simulink model "Transformation_V11"  (R2018a)
settings: Solver=FixedStepDiscrete  StartTime=0.0  StopTime=10.0  RelTol=1e-3
InitFcn:
  | Ts_xadc = 0.1;
values from neighbouring files (symbols this model uses):
  T_mech = 2e-08    [TransformationSkript.m]
libraries: hdlsllib x14, simulink x8, simulink_need_slupdate x1
(part 1 of 4)
settings Model: DataTypeOverride=Off  Creator=trichte  LastModifiedBy=Wendel
settings DataIOCC: LimitDataPoints=on  SaveFormat=Array  SaveOutput=off  SaveTime=off
settings OptimizationCC: BlockReduction=off  ConditionallyExecuteInputs=off  DefaultParameterBehavior=Inlined  LifeSpan=inf
settings DebuggingCC: AlgebraicLoopMsg=error  SolverPrmCheckMsg=warning  SingleTaskRateTransMsg=error  AllowSymbolicDim=off  StrictBusMsg=ErrorOnBusTreatedAsVector  SFUnexpectedBacktrackingDiag=warning  SFNoUnconditionalDefaultTransitionDiag=warning  SFExecutionAtInitializationDiag=none
settings HardwareCC: ProdBitPerPointer=32  ProdBitPerSizeT=32  ProdBitPerPtrDiffT=32  ProdLargestAtomicFloat=None  ProdIntDivRoundTo=Undefined  ProdEndianess=Unspecified  ProdWordSize=32  ProdHWDeviceType=ASIC/FPGA->ASIC/FPGA  ProdEqTarget=off
settings ModelReferenceCC: PropagateSignalLabelsOutOfModel=off
settings CodeAppCC: StateflowObjectComments=on
settings GRTTargetCC: TargetLangStandard=C89/C90 (ANSI)  GeneratePreprocessorConditionals=Disable all
settings ConfigComp: CovMetricSettings=dw  CovHtmlReporting=on  CovSaveCumulativeToWorkspaceVar=on  CovSaveSingleToWorkspaceVar=on  CovExternalEMLEnable=off  CovSFcnEnable=off

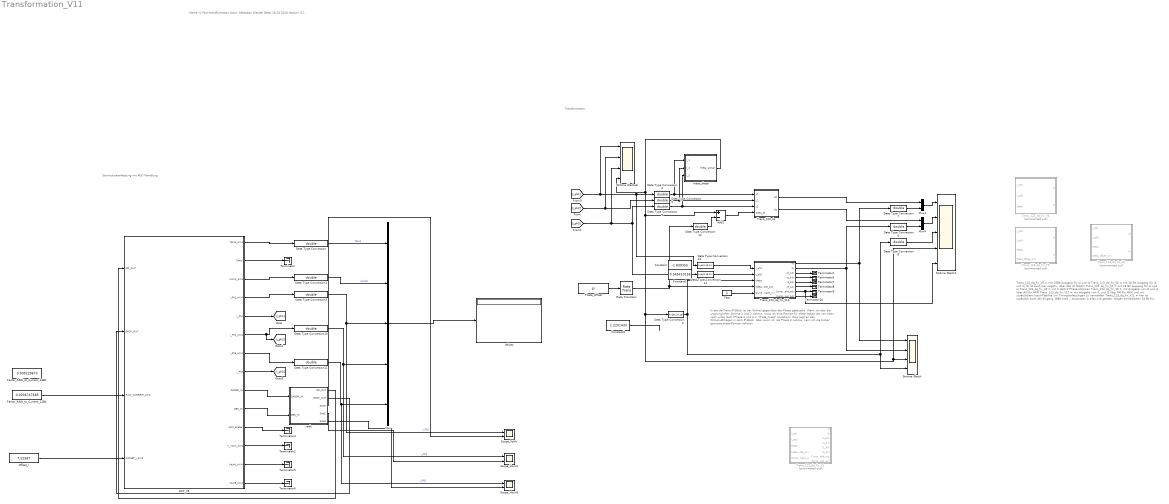
== system Transformation_V11 ==
  note: Trans_123_dq_fix_V5 = mit 16Bit Ausgang für id und iq
      | Trans_123_dq_fix_V6 = mit 18 Bit Ausgang für id und iq (iq ist auch hier negativ, aber das ist falsch)
      | Trans_123_dq_fix_V7 = mit 18 Bit Ausgang für id und iq
      | Trans_123_dq_fix_V8 = mit 3 statt 2 Phasenströmen
      | Trans_123_dq_fix_V9 = mit Ausgabe von id und iq über AXI für ARM
      | Trans_123_dq_fix_V10 = mit Ausgabe von i1 und i3 über AXI für ARM und mit zusätzlichem Input-Pipeline um Timingverletzungen zu vermeiden
      | Trans_123_dq_fix_V11 = hier ist zusätzlich auch der Eingang 18Bit breit
      |
      | ...ansonsten is alles wie gehabt. Wegen einheitlichen 18 Bit für alle Größem wird jedoch 18 Bit genutzt!
  note: Stromistwererfassung mit ADC-Wandlung
  note: Transformation
  note: In der dq-Trans-IP-Block ist der Winkel gegenüber der Phase getauscht.
      | Wenn ich also die ursprünglichen Ströme 1 und 2 nehme,
      |  muss ich eine Rampe für theta haben die von oben nach unten läuft
      | (Phase 2 und 3 in "theta_meas" tauschen).
      | Dies liegt an den Winkel-Abfragen in dem IP-Block.
      | Aber wenn ich die Phase 3 nehme, kann ich die bisher genutzte theta-Rampe nehmen.
  note: Clarke- & Park-transformation
      |
      | Autor: Sebastian Wendel
      | Date: 26.03.2018
      | Version: 0.1
  Add1 : Sum  Inputs=+-  OutDataTypeStr=Inherit: Same as accumulator
  Constant : Constant  Value=-1.839355
  Constant1 : Constant  Value=0.545410156
  Constant2 : Constant  Value=1.2201433
  DUT_V5 : Subsystem  TreatAsAtomicUnit=on
  Data Type Conversion{,1,3..12} (12 alike) : DataTypeConversion  OutDataTypeStr=double
  Data Type Conversion13 : DataTypeConversion  OutDataTypeStr=fixdt(1,18,11)
  Data Type Conversion14 : DataTypeConversion  OutDataTypeStr=fixdt(1,18,11)
  Data Type Conversion2 : DataTypeConversion  OutDataTypeStr=fixdt(1,24,20)
  Factor_RAW_to_Current_12Bit : Constant  Value=0.0036747685  OutDataTypeStr=fixdt(0,24,24)
  Factor_RAW_to_Current_16Bit : Constant  Value=0.000229673  OutDataTypeStr=fixdt(0,24,24)
  Mux : Mux  Inputs=5
  Mux3 : Mux  Inputs=2
  Mux4 : Mux  Inputs=2
  Offset_i : Constant  Value=7.52587  OutDataTypeStr=fixdt(0,16,11)
  Rate Transition : RateTransition  OutPortSampleTime=T_mech
  Scope_Vaux0 : Scope  NumInputPorts=2
  Scope_Vaux8 : Scope  NumInputPorts=2
  Scope_VpVn : Scope  NumInputPorts=2
  Ströme Gleich : Scope  NumInputPorts=4
  Ströme Gleich1 : Scope  NumInputPorts=5
  Ströme Wechsel : Scope  NumInputPorts=4
  Terminator{,1..10} (11 alike) : Terminator
  Test : Constant  OutDataTypeStr=boolean  SampleTime=T_mech
  Theta_Offset : Constant  Value=pi  OutDataTypeStr=fixdt(1,24,20)
  Trans_123_dq : Subsystem
  Trans_123_dq_fix_V1 : Subsystem  Commented=on  TreatAsAtomicUnit=on
  Trans_123_dq_fix_V11 : Subsystem  TreatAsAtomicUnit=on
  Trans_123_dq_fix_V3 : Subsystem  Commented=on  TreatAsAtomicUnit=on
  Trans_123_dq_fix_V5 : Subsystem  Commented=on  TreatAsAtomicUnit=on
  Trans_123_dq_fix_V6 : Subsystem  Commented=on  TreatAsAtomicUnit=on
  Values : Display
      settings: Format=hex (Stored Integer)
  meas_theta : Subsystem
  xadc : Subsystem
  wires:
  DUT_V5/1(Temp_AXI4) -> Data Type Conversion/1
  DUT_V5/3(VccInt_AXI4) -> Data Type Conversion1/1
  DUT_V5/4(i_Ph1_AXI4) -> Data Type Conversion3/1
  DUT_V5/7(i_Ph3_AXI4) -> Data Type Conversion11/1
  DUT_V5/6(i_Ph2_AXI4) -> [i_ph2], Data Type Conversion10/1
  Mux/1 -> Values/1
  Data Type Conversion/1 -> Mux/1  "Temp"
  Data Type Conversion3/1 -> Scope_VpVn/1, Mux/3  "i_Ph1"
  Data Type Conversion10/1 -> Scope_Vaux0/1, Mux/4  "i_Ph2"
  Data Type Conversion11/1 -> Scope_Vaux8/1, Mux/5  "i_Ph3"
  Data Type Conversion1/1 -> Mux/2  "VccInt"
  DUT_V5/9(DADDR_IN) -> xadc/1(DADDR_IN)
  DUT_V5/10(DEN_IN) -> xadc/2(DEN_IN)
  xadc/2(DRDY_OUT) -> DUT_V5/2(DRDY_OUT)
  xadc/1(DO_OUT) -> DUT_V5/1(DO_OUT)
  DUT_V5/2(Temp) -> Terminator/1
  DUT_V5/11(ADC_enable) -> Terminator4/1
  Factor_RAW_to_Current_12Bit/1 -> DUT_V5/3(RAW_CURRENT_AXI4)
  Offset_i/1 -> DUT_V5/4(OFFSET_I_AXI4)
  DUT_V5/12(V_VpVn_AXI4) -> Terminator2/1
  DUT_V5/13(Vaux0_AXI4) -> Terminator5/1
  DUT_V5/14(Vaux8_AXI4) -> Terminator6/1
  xadc/3(Sine1) -> Scope_VpVn/2
  xadc/4(Sine2) -> Scope_Vaux0/2
  xadc/5(Sine3) -> Scope_Vaux8/2
  Data Type Conversion2/1 -> Trans_123_dq_fix_V11/3(theta), Ströme Gleich/4, Data Type Conversion8/1
  Trans_123_dq/1(Ud) -> Mux3/1
  Trans_123_dq/2(Uq) -> Mux4/1
  Mux3/1 -> Ströme Gleich1/1
  Data Type Conversion7/1 -> Mux3/2
  Data Type Conversion6/1 -> Mux4/2
  Mux4/1 -> Ströme Gleich1/2
  Data Type Conversion8/1 -> Ströme Gleich1/3
  meas_theta/1(theta_arctan) -> Ströme Wechsel/4, Data Type Conversion2/1, Ströme Gleich/3, Ströme Gleich1/4, Add1/1
  Data Type Conversion4/1 -> meas_theta/1(I_1), Trans_123_dq/1(L1)
  Data Type Conversion9/1 -> meas_theta/3(I_3), Trans_123_dq/3(L3)
  Data Type Conversion5/1 -> meas_theta/2(I_2), Trans_123_dq/2(L2)
  DUT_V5/5(i_Ph1) -> [i_ph1]
  DUT_V5/8(i_Ph3) -> [i_ph3]
  [i_ph2] -> Ströme Wechsel/2, Data Type Conversion5/1
  Trans_123_dq_fix_V11/1(id) -> Ströme Gleich/1, Data Type Conversion7/1
  Trans_123_dq_fix_V11/2(iq) -> Ströme Gleich/2, Data Type Conversion6/1
  Theta_Offset/1 -> Rate Transition/1
  Data Type Conversion12/1 -> Add1/2
  Add1/1 -> Trans_123_dq/4(theta_el)
  Trans_123_dq_fix_V11/4(iq_AXI) -> Terminator3/1
  Trans_123_dq_fix_V11/3(id_AXI) -> Terminator1/1
  Rate Transition/1 -> Data Type Conversion12/1, Trans_123_dq_fix_V11/4(theta_offset_AXI)
  Trans_123_dq_fix_V11/5(i1_AXI) -> Terminator7/1
  Trans_123_dq_fix_V11/6(i3_AXI) -> Terminator8/1
  Data Type Conversion13/1 -> Trans_123_dq_fix_V11/1(i_ph1)
  Data Type Conversion14/1 -> Trans_123_dq_fix_V11/2(i_ph3)
  Trans_123_dq_fix_V11/7(CurrentValid_out) -> Ströme Gleich1/5, Terminator9/1
  Test/1 -> Trans_123_dq_fix_V11/5(CurrentValid_in)
  Trans_123_dq_fix_V11/8(CurrentValid_out_AXI) -> Terminator10/1
  [i_ph1] -> Ströme Wechsel/1, Data Type Conversion13/1, Data Type Conversion4/1
  [i_ph3] -> Ströme Wechsel/3, Data Type Conversion14/1, Data Type Conversion9/1
  Constant2/1 -> ?

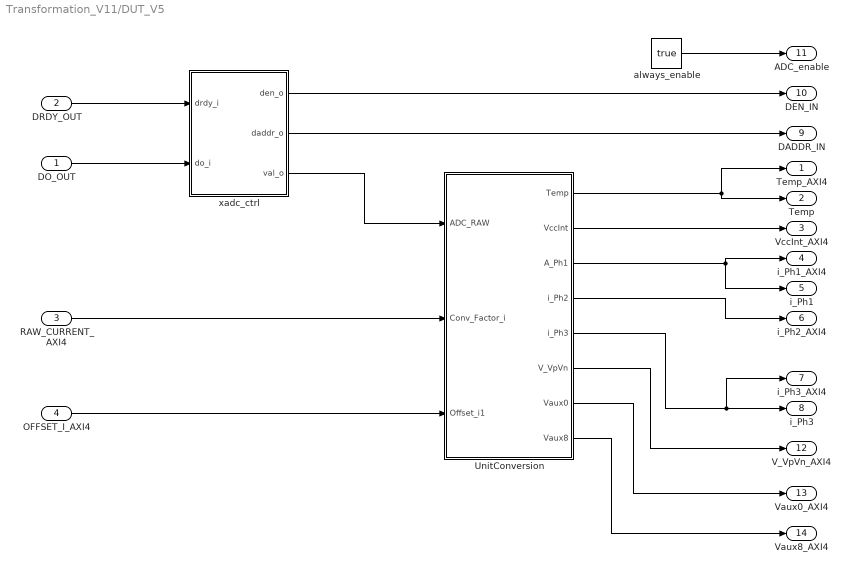
== system Transformation_V11/DUT_V5 ==
  DO_OUT : Inport
  DRDY_OUT : Inport  Port=2
  RAW_CURRENT_AXI4 : Inport  Port=3
  OFFSET_I_AXI4 : Inport  Port=4
  UnitConversion : Subsystem
  always_enable : Constant  Value=true  OutDataTypeStr=boolean
  xadc_ctrl : MATLAB Function  TreatAsAtomicUnit=on
  Temp_AXI4 : Outport
  Temp : Outport  Port=2
  VccInt_AXI4 : Outport  Port=3
  i_Ph1_AXI4 : Outport  Port=4
  i_Ph1 : Outport  Port=5
  i_Ph2_AXI4 : Outport  Port=6
  i_Ph3_AXI4 : Outport  Port=7
  i_Ph3 : Outport  Port=8
  DADDR_IN : Outport  Port=9
  DEN_IN : Outport  Port=10
  ADC_enable : Outport  Port=11
  V_VpVn_AXI4 : Outport  Port=12
  Vaux0_AXI4 : Outport  Port=13
  Vaux8_AXI4 : Outport  Port=14
  wires:
  xadc_ctrl/3(val_o) -> UnitConversion/1(ADC_RAW)
  UnitConversion/5(i_Ph3) -> i_Ph3/1, i_Ph3_AXI4/1
  UnitConversion/3(A_Ph1) -> i_Ph1/1, i_Ph1_AXI4/1
  UnitConversion/4(i_Ph2) -> i_Ph2_AXI4/1
  UnitConversion/2(VccInt) -> VccInt_AXI4/1
  UnitConversion/1(Temp) -> Temp/1, Temp_AXI4/1
  DRDY_OUT/1 -> xadc_ctrl/1(drdy_i)
  DO_OUT/1 -> xadc_ctrl/2(do_i)
  xadc_ctrl/1(den_o) -> DEN_IN/1
  xadc_ctrl/2(daddr_o) -> DADDR_IN/1
  always_enable/1 -> ADC_enable/1
  RAW_CURRENT_AXI4/1 -> UnitConversion/2(Conv_Factor_i)
  UnitConversion/6(V_VpVn) -> V_VpVn_AXI4/1
  OFFSET_I_AXI4/1 -> UnitConversion/3(Offset_i1)
  UnitConversion/7(Vaux0) -> Vaux0_AXI4/1
  UnitConversion/8(Vaux8) -> Vaux8_AXI4/1

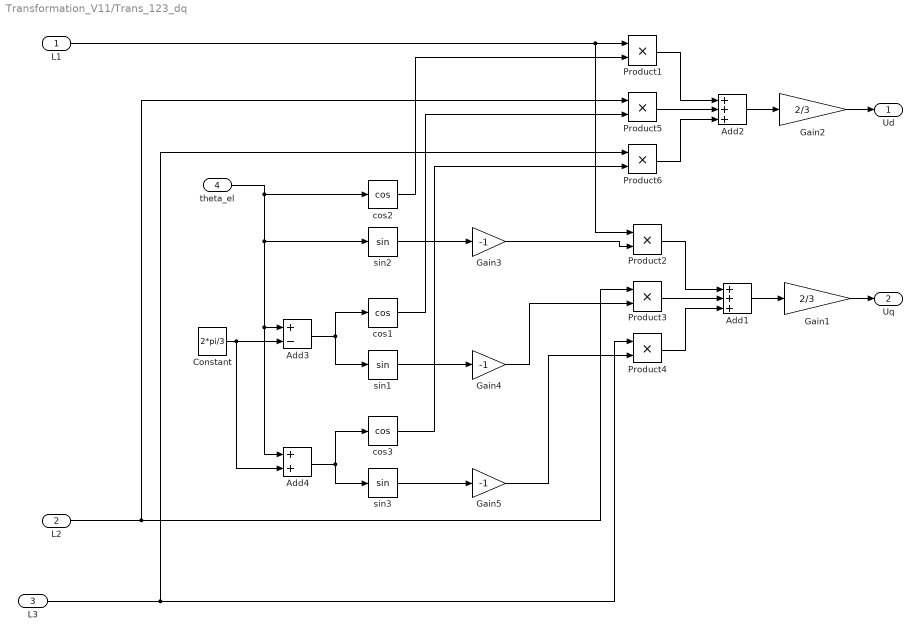
== system Transformation_V11/Trans_123_dq ==
  L1 : Inport
  L2 : Inport  Port=2
  L3 : Inport  Port=3
  theta_el : Inport  Port=4
  Add1 : Sum  Inputs=+++
  Add2 : Sum  Inputs=+++
  Add3 : Sum  Inputs=+-
  Add4 : Sum
  Constant : Constant  Value=2*pi/3  SampleTime=T_mech
  Gain1 : Gain  Gain=2/3
  Gain2 : Gain  Gain=2/3
  Gain3 : Gain  Gain=-1
  Gain4 : Gain  Gain=-1
  Gain5 : Gain  Gain=-1
  Product{1..6} (6 alike) : Product  RndMeth=Zero
  cos1 : Trigonometry  Operator=cos
  cos2 : Trigonometry  Operator=cos
  cos3 : Trigonometry  Operator=cos
  sin1 : Trigonometry
  sin2 : Trigonometry
  sin3 : Trigonometry
  Ud : Outport
  Uq : Outport  Port=2
  wires:
  Gain5/1 -> Product4/2
  Gain4/1 -> Product3/2
  Gain3/1 -> Product2/2
  sin3/1 -> Gain5/1
  sin1/1 -> Gain4/1
  sin2/1 -> Gain3/1
  L3/1 -> Product4/1, Product6/1
  L2/1 -> Product3/1, Product5/1
  L1/1 -> Product2/1, Product1/1
  Gain1/1 -> Uq/1
  Gain2/1 -> Ud/1
  Product6/1 -> Add2/3
  Add2/1 -> Gain2/1
  Product5/1 -> Add2/2
  Product4/1 -> Add1/3
  Add1/1 -> Gain1/1
  Product2/1 -> Add1/1
  Product3/1 -> Add1/2
  theta_el/1 -> cos2/1, Add3/1, Add4/1, sin2/1
  Constant/1 -> Add3/2, Add4/2
  Add3/1 -> cos1/1, sin1/1
  Add4/1 -> cos3/1, sin3/1
  Product1/1 -> Add2/1
  cos3/1 -> Product6/2
  cos1/1 -> Product5/2
  cos2/1 -> Product1/2

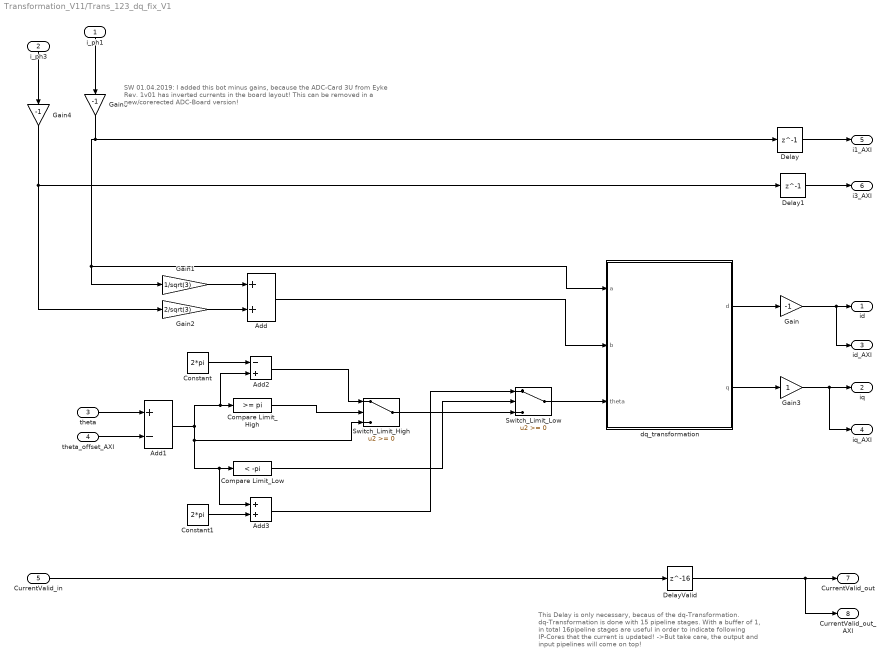
== system Transformation_V11/Trans_123_dq_fix_V1 ==
  note: This Delay is only necessary, becaus of the dq-Transformation.
      | dq-Transformation is done with 15 pipeline stages.
      | With a buffer of 1, in total 16pipeline stages are useful in order to
      |  indicate following IP-Cores that the current is updated!
      | ->But take care, the output and input pipelines will come on top!
  note: SW 01.04.2019: I added this bot minus gains, because the ADC-Card 3U from
      | Eyke Rev. 1v01 has inverted currents in the board layout!
      | This can be removed in a new/corerected ADC-Board version!
  i_ph1 : Inport
  i_ph3 : Inport  Port=2
  theta : Inport  Port=3
  theta_offset_AXI : Inport  Port=4
  CurrentValid_in : Inport  Port=5
  Add : Sum
  Add1 : Sum  Inputs=+-  OutDataTypeStr=Inherit: Same as accumulator
  Add2 : Sum  Inputs=-+  OutDataTypeStr=Inherit: Same as first input
  Add3 : Sum  OutDataTypeStr=Inherit: Same as first input
  Compare Limit_High : simulink/Logic and Bit Operations/Compare To Constant  relop=>=  const=pi  OutDataTypeStr=boolean
  Compare Limit_Low : simulink/Logic and Bit Operations/Compare To Constant  relop=<  const=-pi  OutDataTypeStr=boolean
  Constant : Constant  Value=2*pi  OutDataTypeStr=fixdt(1,24,20)  SampleTime=-1
  Constant1 : Constant  Value=2*pi  OutDataTypeStr=fixdt(1,24,20)  SampleTime=-1
  Delay : Delay  DelayLength=1
  Delay1 : Delay  DelayLength=1
  DelayValid : Delay  DelayLength=16
  Gain : Gain  Gain=-1  OutDataTypeStr=fixdt(1,18,11)
  Gain1 : Gain  Gain=1/sqrt(3)  OutDataTypeStr=Inherit: Same as input
  Gain2 : Gain  Gain=2/sqrt(3)  OutDataTypeStr=Inherit: Same as input
  Gain3 : Gain  OutDataTypeStr=fixdt(1,18,11)
  Gain4 : Gain  Gain=-1  OutDataTypeStr=fixdt(1,18,11)
  Gain6 : Gain  Gain=-1  OutDataTypeStr=fixdt(1,18,11)
  Switch_Limit_High : Switch  OutDataTypeStr=fixdt(1,24,20)
  Switch_Limit_Low : Switch  OutDataTypeStr=fixdt(1,24,20)
  dq_transformation : MATLAB Function  TreatAsAtomicUnit=on
  id : Outport
  iq : Outport  Port=2
  id_AXI : Outport  Port=3
  iq_AXI : Outport  Port=4
  i1_AXI : Outport  Port=5
  i3_AXI : Outport  Port=6
  CurrentValid_out : Outport  Port=7
  CurrentValid_out_AXI : Outport  Port=8
  wires:
  Add/1 -> dq_transformation/2(b)
  Gain1/1 -> Add/1
  Gain2/1 -> Add/2
  dq_transformation/2(q) -> Gain3/1
  dq_transformation/1(d) -> Gain/1
  theta/1 -> Add1/1
  Add1/1 -> Switch_Limit_High/3, Add3/1, Compare Limit_Low/1, Add2/2, Compare Limit_High/1
  theta_offset_AXI/1 -> Add1/2
  Switch_Limit_Low/1 -> dq_transformation/3(theta)
  Switch_Limit_High/1 -> Switch_Limit_Low/3
  Compare Limit_High/1 -> Switch_Limit_High/2
  Compare Limit_Low/1 -> Switch_Limit_Low/2
  Constant/1 -> Add2/1
  Add2/1 -> Switch_Limit_High/1
  Constant1/1 -> Add3/2
  Add3/1 -> Switch_Limit_Low/1
  Gain3/1 -> iq_AXI/1, iq/1
  Gain/1 -> id_AXI/1, id/1
  Delay/1 -> i1_AXI/1
  Delay1/1 -> i3_AXI/1
  i_ph3/1 -> Gain4/1
  i_ph1/1 -> Gain6/1
  DelayValid/1 -> CurrentValid_out_AXI/1, CurrentValid_out/1
  CurrentValid_in/1 -> DelayValid/1
  Gain6/1 -> Gain1/1, dq_transformation/1(a), Delay/1
  Gain4/1 -> Gain2/1, Delay1/1

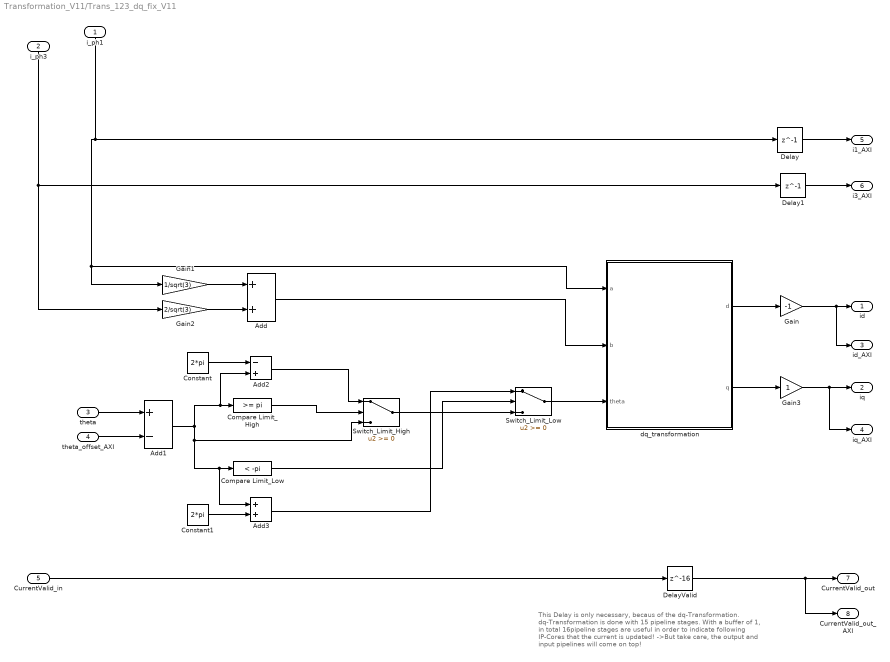
== system Transformation_V11/Trans_123_dq_fix_V11 ==
  note: This Delay is only necessary, becaus of the dq-Transformation.
      | dq-Transformation is done with 15 pipeline stages.
      | With a buffer of 1, in total 16pipeline stages are useful in order to
      |  indicate following IP-Cores that the current is updated!
      | ->But take care, the output and input pipelines will come on top!
  i_ph1 : Inport
  i_ph3 : Inport  Port=2
  theta : Inport  Port=3
  theta_offset_AXI : Inport  Port=4
  CurrentValid_in : Inport  Port=5
  Add : Sum
  Add1 : Sum  Inputs=+-  OutDataTypeStr=Inherit: Same as accumulator
  Add2 : Sum  Inputs=-+  OutDataTypeStr=Inherit: Same as first input
  Add3 : Sum  OutDataTypeStr=Inherit: Same as first input
  Compare Limit_High : simulink/Logic and Bit Operations/Compare To Constant  relop=>=  const=pi  OutDataTypeStr=boolean
  Compare Limit_Low : simulink/Logic and Bit Operations/Compare To Constant  relop=<  const=-pi  OutDataTypeStr=boolean
  Constant : Constant  Value=2*pi  OutDataTypeStr=fixdt(1,24,20)  SampleTime=-1
  Constant1 : Constant  Value=2*pi  OutDataTypeStr=fixdt(1,24,20)  SampleTime=-1
  Delay : Delay  DelayLength=1
  Delay1 : Delay  DelayLength=1
  DelayValid : Delay  DelayLength=16
  Gain : Gain  Gain=-1  OutDataTypeStr=fixdt(1,18,11)
  Gain1 : Gain  Gain=1/sqrt(3)  OutDataTypeStr=Inherit: Same as input
  Gain2 : Gain  Gain=2/sqrt(3)  OutDataTypeStr=Inherit: Same as input
  Gain3 : Gain  OutDataTypeStr=fixdt(1,18,11)
  Switch_Limit_High : Switch  OutDataTypeStr=fixdt(1,24,20)
  Switch_Limit_Low : Switch  OutDataTypeStr=fixdt(1,24,20)
  dq_transformation : MATLAB Function  TreatAsAtomicUnit=on
  id : Outport
  iq : Outport  Port=2
  id_AXI : Outport  Port=3
  iq_AXI : Outport  Port=4
  i1_AXI : Outport  Port=5
  i3_AXI : Outport  Port=6
  CurrentValid_out : Outport  Port=7
  CurrentValid_out_AXI : Outport  Port=8
  wires:
  Add/1 -> dq_transformation/2(b)
  Gain1/1 -> Add/1
  Gain2/1 -> Add/2
  dq_transformation/2(q) -> Gain3/1
  dq_transformation/1(d) -> Gain/1
  theta/1 -> Add1/1
  Add1/1 -> Switch_Limit_High/3, Add3/1, Compare Limit_Low/1, Add2/2, Compare Limit_High/1
  theta_offset_AXI/1 -> Add1/2
  Switch_Limit_Low/1 -> dq_transformation/3(theta)
  Switch_Limit_High/1 -> Switch_Limit_Low/3
  Compare Limit_High/1 -> Switch_Limit_High/2
  Compare Limit_Low/1 -> Switch_Limit_Low/2
  Constant/1 -> Add2/1
  Add2/1 -> Switch_Limit_High/1
  Constant1/1 -> Add3/2
  Add3/1 -> Switch_Limit_Low/1
  Gain3/1 -> iq_AXI/1, iq/1
  Gain/1 -> id_AXI/1, id/1
  Delay/1 -> i1_AXI/1
  Delay1/1 -> i3_AXI/1
  DelayValid/1 -> CurrentValid_out_AXI/1, CurrentValid_out/1
  CurrentValid_in/1 -> DelayValid/1
  i_ph1/1 -> Gain1/1, dq_transformation/1(a), Delay/1
  i_ph3/1 -> Gain2/1, Delay1/1

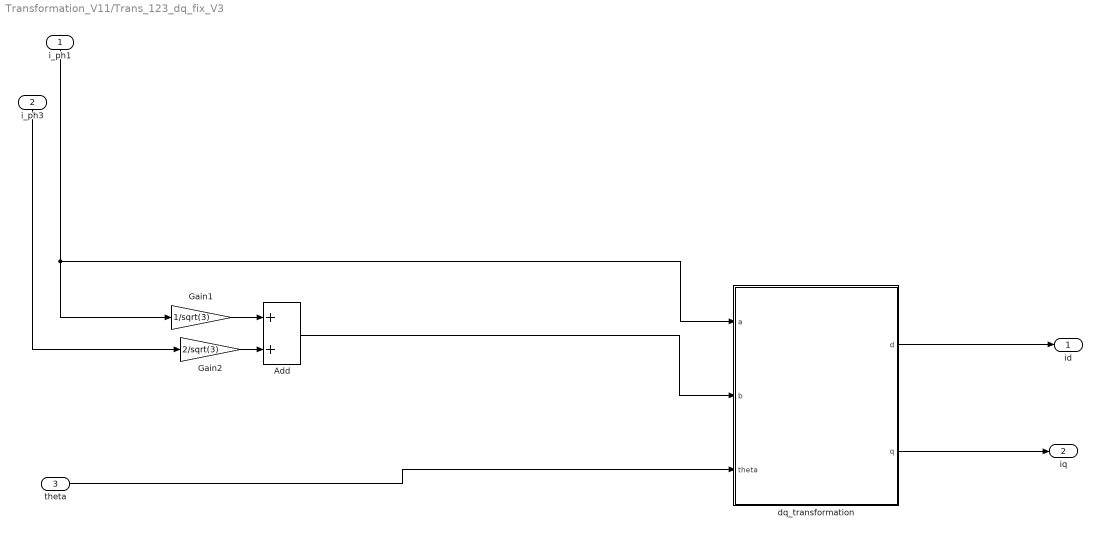
== system Transformation_V11/Trans_123_dq_fix_V3 ==
  i_ph1 : Inport
  i_ph3 : Inport  Port=2
  theta : Inport  Port=3
  Add : Sum
  Gain1 : Gain  Gain=1/sqrt(3)  OutDataTypeStr=Inherit: Same as input
  Gain2 : Gain  Gain=2/sqrt(3)  OutDataTypeStr=Inherit: Same as input
  dq_transformation : MATLAB Function  TreatAsAtomicUnit=on
  id : Outport
  iq : Outport  Port=2
  wires:
  i_ph1/1 -> dq_transformation/1(a), Gain1/1
  Add/1 -> dq_transformation/2(b)
  Gain1/1 -> Add/1
  Gain2/1 -> Add/2
  dq_transformation/2(q) -> iq/1
  dq_transformation/1(d) -> id/1
  i_ph3/1 -> Gain2/1
  theta/1 -> dq_transformation/3(theta)

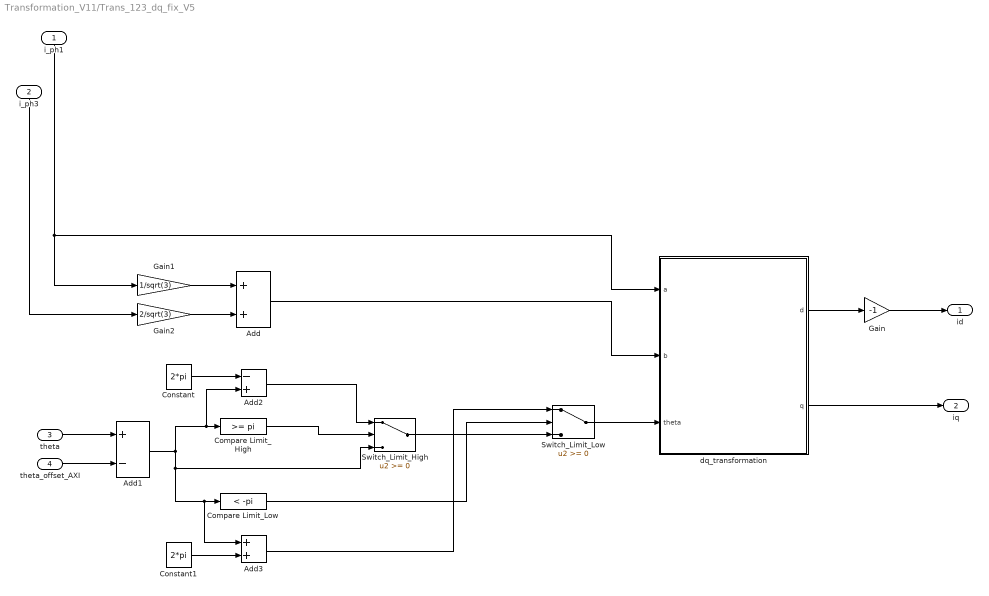
== system Transformation_V11/Trans_123_dq_fix_V5 ==
  i_ph1 : Inport
  i_ph3 : Inport  Port=2
  theta : Inport  Port=3
  theta_offset_AXI : Inport  Port=4
  Add : Sum
  Add1 : Sum  Inputs=+-  OutDataTypeStr=Inherit: Same as accumulator
  Add2 : Sum  Inputs=-+  OutDataTypeStr=Inherit: Same as first input
  Add3 : Sum  OutDataTypeStr=Inherit: Same as first input
  Compare Limit_High : simulink/Logic and Bit Operations/Compare To Constant  relop=>=  const=pi  OutDataTypeStr=boolean
  Compare Limit_Low : simulink/Logic and Bit Operations/Compare To Constant  relop=<  const=-pi  OutDataTypeStr=boolean
  Constant : Constant  Value=2*pi  OutDataTypeStr=fixdt(1,24,20)  SampleTime=-1
  Constant1 : Constant  Value=2*pi  OutDataTypeStr=fixdt(1,24,20)  SampleTime=-1
  Gain : Gain  Gain=-1  OutDataTypeStr=Inherit: Same as input
  Gain1 : Gain  Gain=1/sqrt(3)  OutDataTypeStr=Inherit: Same as input
  Gain2 : Gain  Gain=2/sqrt(3)  OutDataTypeStr=Inherit: Same as input
  Switch_Limit_High : Switch  OutDataTypeStr=fixdt(1,24,20)
  Switch_Limit_Low : Switch  OutDataTypeStr=fixdt(1,24,20)
  dq_transformation : MATLAB Function  TreatAsAtomicUnit=on
  id : Outport
  iq : Outport  Port=2
  wires:
  i_ph1/1 -> dq_transformation/1(a), Gain1/1
  Add/1 -> dq_transformation/2(b)
  Gain1/1 -> Add/1
  Gain2/1 -> Add/2
  dq_transformation/2(q) -> iq/1
  dq_transformation/1(d) -> Gain/1
  i_ph3/1 -> Gain2/1
  theta/1 -> Add1/1
  Add1/1 -> Switch_Limit_High/3, Add3/1, Compare Limit_Low/1, Add2/2, Compare Limit_High/1
  theta_offset_AXI/1 -> Add1/2
  Switch_Limit_Low/1 -> dq_transformation/3(theta)
  Switch_Limit_High/1 -> Switch_Limit_Low/3
  Compare Limit_High/1 -> Switch_Limit_High/2
  Compare Limit_Low/1 -> Switch_Limit_Low/2
  Constant/1 -> Add2/1
  Add2/1 -> Switch_Limit_High/1
  Constant1/1 -> Add3/2
  Add3/1 -> Switch_Limit_Low/1
  Gain/1 -> id/1

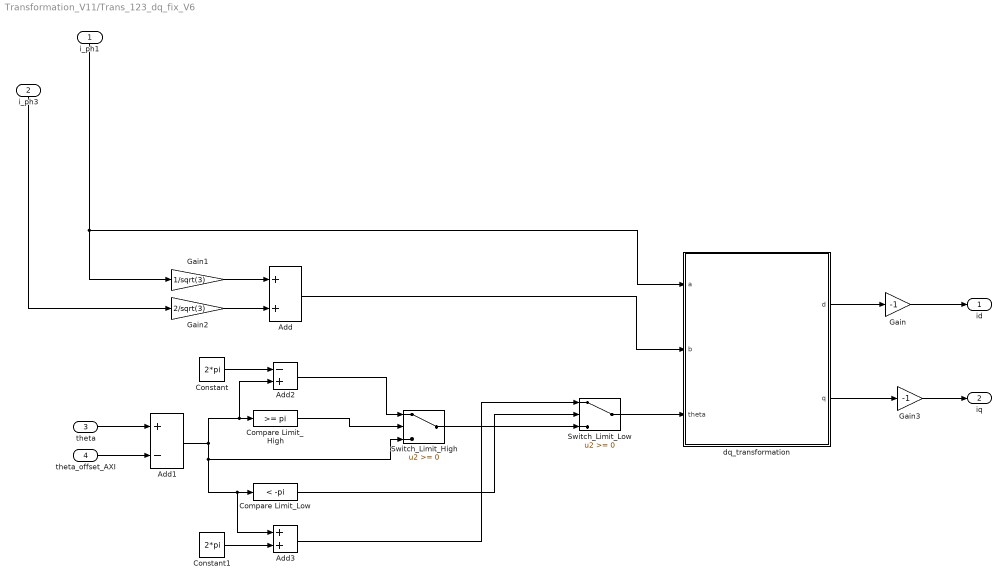
== system Transformation_V11/Trans_123_dq_fix_V6 ==
  i_ph1 : Inport
  i_ph3 : Inport  Port=2
  theta : Inport  Port=3
  theta_offset_AXI : Inport  Port=4
  Add : Sum
  Add1 : Sum  Inputs=+-  OutDataTypeStr=Inherit: Same as accumulator
  Add2 : Sum  Inputs=-+  OutDataTypeStr=Inherit: Same as first input
  Add3 : Sum  OutDataTypeStr=Inherit: Same as first input
  Compare Limit_High : simulink/Logic and Bit Operations/Compare To Constant  relop=>=  const=pi  OutDataTypeStr=boolean
  Compare Limit_Low : simulink/Logic and Bit Operations/Compare To Constant  relop=<  const=-pi  OutDataTypeStr=boolean
  Constant : Constant  Value=2*pi  OutDataTypeStr=fixdt(1,24,20)  SampleTime=-1
  Constant1 : Constant  Value=2*pi  OutDataTypeStr=fixdt(1,24,20)  SampleTime=-1
  Gain : Gain  Gain=-1  OutDataTypeStr=fixdt(1,18,11)
  Gain1 : Gain  Gain=1/sqrt(3)  OutDataTypeStr=Inherit: Same as input
  Gain2 : Gain  Gain=2/sqrt(3)  OutDataTypeStr=Inherit: Same as input
  Gain3 : Gain  Gain=-1  OutDataTypeStr=fixdt(1,18,11)
  Switch_Limit_High : Switch  OutDataTypeStr=fixdt(1,24,20)
  Switch_Limit_Low : Switch  OutDataTypeStr=fixdt(1,24,20)
  dq_transformation : MATLAB Function  TreatAsAtomicUnit=on
  id : Outport
  iq : Outport  Port=2
  wires:
  i_ph1/1 -> dq_transformation/1(a), Gain1/1
  Add/1 -> dq_transformation/2(b)
  Gain1/1 -> Add/1
  Gain2/1 -> Add/2
  dq_transformation/2(q) -> Gain3/1
  dq_transformation/1(d) -> Gain/1
  i_ph3/1 -> Gain2/1
  theta/1 -> Add1/1
  Add1/1 -> Switch_Limit_High/3, Add3/1, Compare Limit_Low/1, Add2/2, Compare Limit_High/1
  theta_offset_AXI/1 -> Add1/2
  Switch_Limit_Low/1 -> dq_transformation/3(theta)
  Switch_Limit_High/1 -> Switch_Limit_Low/3
  Compare Limit_High/1 -> Switch_Limit_High/2
  Compare Limit_Low/1 -> Switch_Limit_Low/2
  Constant/1 -> Add2/1
  Add2/1 -> Switch_Limit_High/1
  Constant1/1 -> Add3/2
  Add3/1 -> Switch_Limit_Low/1
  Gain/1 -> id/1
  Gain3/1 -> iq/1

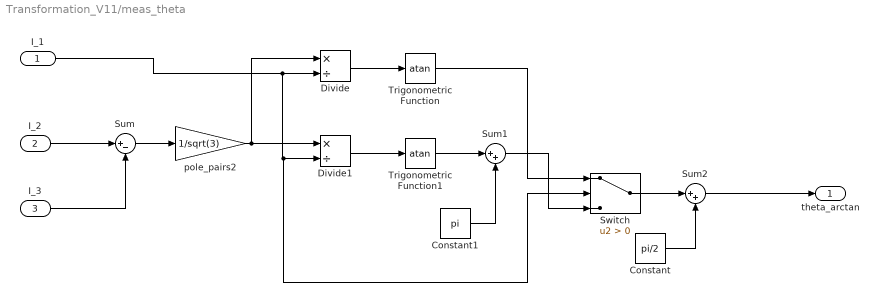
== system Transformation_V11/meas_theta ==
  I_1 : Inport
  I_2 : Inport  Port=2
  I_3 : Inport  Port=3
  Constant : Constant  Value=pi/2
  Constant1 : Constant  Value=pi
  Divide : Product  Inputs=*/
  Divide1 : Product  Inputs=*/
  Sum : Sum  Inputs=|+-
  Sum1 : Sum  Inputs=|++
  Sum2 : Sum  Inputs=|++
  Switch : Switch  Criteria=u2 > Threshold
  Trigonometric Function : Trigonometry  Operator=atan
  Trigonometric Function1 : Trigonometry  Operator=atan
  pole_pairs2 : Gain  Gain=1/sqrt(3)
  theta_arctan : Outport
  wires:
  Divide/1 -> Trigonometric Function/1
  Divide1/1 -> Trigonometric Function1/1
  Trigonometric Function1/1 -> Sum1/1
  pole_pairs2/1 -> Divide/1, Divide1/1
  Sum/1 -> pole_pairs2/1
  I_3/1 -> Sum/2
  I_2/1 -> Sum/1
  I_1/1 -> Switch/2, Divide1/2, Divide/2
  Sum1/1 -> Switch/3
  Trigonometric Function/1 -> Switch/1
  Switch/1 -> Sum2/1
  Constant/1 -> Sum2/2
  Constant1/1 -> Sum1/2
  Sum2/1 -> theta_arctan/1

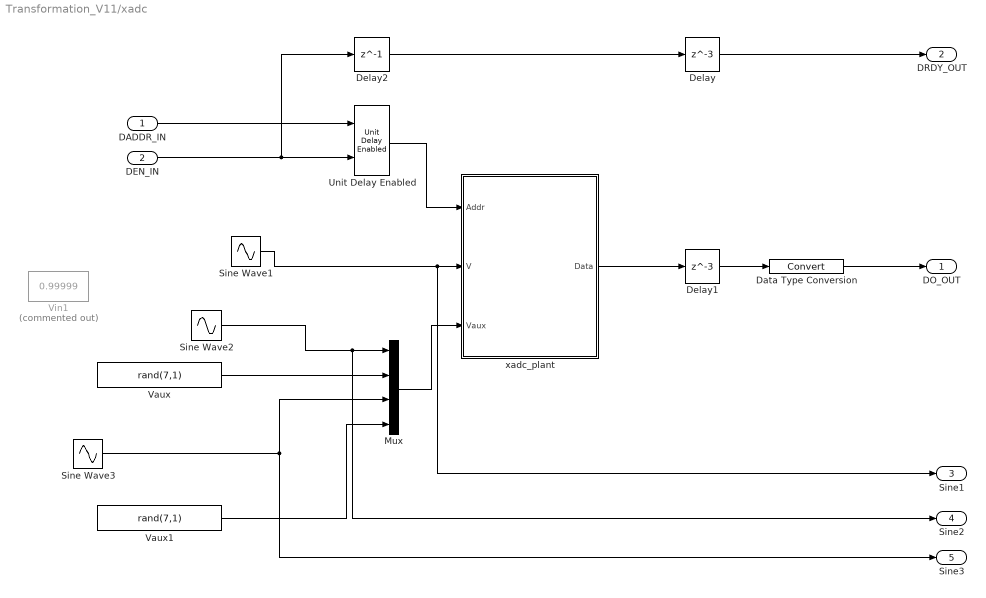
== system Transformation_V11/xadc ==
  DADDR_IN : Inport  OutDataTypeStr=fixdt(0,7,0)
  DEN_IN : Inport  Port=2  OutDataTypeStr=boolean
  Data Type Conversion : DataTypeConversion
  Delay : Delay  DelayLength=3
  Delay1 : Delay  DelayLength=3
  Delay2 : Delay  DelayLength=1
  Mux : Mux
  Sine Wave1 : Sin  Amplitude=0.49  Bias=0.5  Frequency=50  SampleTime=T_mech
  Sine Wave2 : Sin  Amplitude=0.49  Bias=0.5  Frequency=50  Phase=-2*pi/3  SampleTime=T_mech
  Sine Wave3 : Sin  Amplitude=0.49  Bias=0.5  Frequency=50  Phase=2*pi/3  SampleTime=T_mech
  Unit Delay Enabled : simulink_need_slupdate/Unit Delay Enabled  vinit=0.0  tsamp=-1
      settings: SourceProductName=Simulink  SourceProductBaseCode=SL
  Vaux : Constant  Value=rand(7,1)  SampleTime=-1
  Vaux1 : Constant  Value=rand(7,1)  SampleTime=-1
  Vin1 : Constant  Commented=on  Value=0.99999  SampleTime=-1
  xadc_plant : Subsystem
  DO_OUT : Outport  OutDataTypeStr=fixdt(0,16,0)
  DRDY_OUT : Outport  Port=2  OutDataTypeStr=boolean
  Sine1 : Outport  Port=3
  Sine2 : Outport  Port=4
  Sine3 : Outport  Port=5
  wires:
  DEN_IN/1 -> Delay2/1, Unit Delay Enabled/2
  DADDR_IN/1 -> Unit Delay Enabled/1
  Data Type Conversion/1 -> DO_OUT/1
  Delay/1 -> DRDY_OUT/1
  Delay1/1 -> Data Type Conversion/1
  Delay2/1 -> Delay/1
  xadc_plant/1(Data) -> Delay1/1
  Unit Delay Enabled/1 -> xadc_plant/1(Addr)
  Sine Wave1/1 -> Sine1/1, xadc_plant/2(V)
  Vaux/1 -> Mux/2
  Vaux1/1 -> Mux/4
  Sine Wave3/1 -> Mux/3, Sine3/1
  Sine Wave2/1 -> Sine2/1, Mux/1
  Mux/1 -> xadc_plant/3(Vaux)

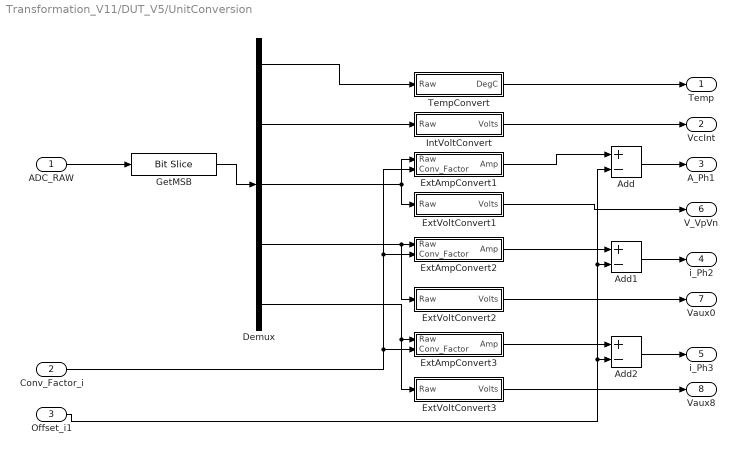
== system Transformation_V11/DUT_V5/UnitConversion ==
  ADC_RAW : Inport
  Conv_Factor_i : Inport  Port=2
  Offset_i1 : Inport  Port=3
  Add : Sum  Inputs=+-  OutDataTypeStr=fixdt(1,16,11)
  Add1 : Sum  Inputs=+-  OutDataTypeStr=fixdt(1,16,11)
  Add2 : Sum  Inputs=+-  OutDataTypeStr=fixdt(1,16,11)
  Demux : Demux  Outputs=5
  ExtAmpConvert1 : Subsystem  TreatAsAtomicUnit=on
  ExtAmpConvert2 : Subsystem  TreatAsAtomicUnit=on
  ExtAmpConvert3 : Subsystem  TreatAsAtomicUnit=on
  ExtVoltConvert1 : Subsystem  TreatAsAtomicUnit=on
  ExtVoltConvert2 : Subsystem  TreatAsAtomicUnit=on
  ExtVoltConvert3 : Subsystem  TreatAsAtomicUnit=on
  GetMSB : hdlsllib/Logic and Bit Operations/Bit Slice  lidx=15  ridx=4
  IntVoltConvert : Subsystem  TreatAsAtomicUnit=on
  TempConvert : Subsystem
  Temp : Outport
  VccInt : Outport  Port=2
  A_Ph1 : Outport  Port=3
  i_Ph2 : Outport  Port=4
  i_Ph3 : Outport  Port=5
  V_VpVn : Outport  Port=6
  Vaux0 : Outport  Port=7
  Vaux8 : Outport  Port=8
  wires:
  ADC_RAW/1 -> GetMSB/1
  GetMSB/1 -> Demux/1
  TempConvert/1(DegC) -> Temp/1
  IntVoltConvert/1(Volts) -> VccInt/1
  ExtAmpConvert1/1(Amp) -> Add/1
  ExtVoltConvert2/1(Volts) -> Vaux0/1
  ExtVoltConvert3/1(Volts) -> Vaux8/1
  Demux/1 -> TempConvert/1(Raw)
  Demux/2 -> IntVoltConvert/1(Raw)
  Demux/3 -> ExtVoltConvert1/1(Raw), ExtAmpConvert1/1(Raw)
  Demux/4 -> ExtVoltConvert2/1(Raw), ExtAmpConvert2/1(Raw)
  Demux/5 -> ExtAmpConvert3/1(Raw), ExtVoltConvert3/1(Raw)
  Conv_Factor_i/1 -> ExtAmpConvert3/2(Conv_Factor), ExtAmpConvert2/2(Conv_Factor), ExtAmpConvert1/2(Conv_Factor)
  ExtVoltConvert1/1(Volts) -> V_VpVn/1
  Add/1 -> A_Ph1/1
  ExtAmpConvert2/1(Amp) -> Add1/1
  Add1/1 -> i_Ph2/1
  ExtAmpConvert3/1(Amp) -> Add2/1
  Add2/1 -> i_Ph3/1
  Offset_i1/1 -> Add2/2, Add/2, Add1/2

== system Transformation_V11/xadc/xadc_plant ==
  Addr : Inport
  V : Inport  Port=2
  Vaux : Inport  Port=3
  AuxChan : Subsystem
  Bit Slice : hdlsllib/Logic and Bit Operations/Bit Slice  lidx=3  ridx=0
  Bit Slice1 : hdlsllib/Logic and Bit Operations/Bit Slice  lidx=4  ridx=4
  IntChan : Subsystem
  Switch : Switch  Criteria=u2 ~= 0
  Data : Outport
  wires:
  Addr/1 -> Bit Slice1/1, Bit Slice/1
  Bit Slice/1 -> IntChan/1(Addr), AuxChan/1(Addr)
  Vaux/1 -> AuxChan/2(Vaux)
  V/1 -> IntChan/2(V)
  Switch/1 -> Data/1
  Bit Slice1/1 -> Switch/2
  IntChan/1(Int_ADC) -> Switch/3
  AuxChan/1(Aux_ADC) -> Switch/1

== system Transformation_V11/DUT_V5/UnitConversion/ExtAmpConvert1 ==
  Raw : Inport
  Conv_Factor : Inport  Port=2
  Product : Product  OutDataTypeStr=fixdt(1,16,11)
  Amp : Outport
  wires:
  Raw/1 -> Product/1
  Product/1 -> Amp/1
  Conv_Factor/1 -> Product/2

== system Transformation_V11/DUT_V5/UnitConversion/ExtAmpConvert2 ==
  Raw : Inport
  Conv_Factor : Inport  Port=2
  Product : Product  OutDataTypeStr=fixdt(1,16,11)
  Amp : Outport
  wires:
  Raw/1 -> Product/1
  Product/1 -> Amp/1
  Conv_Factor/1 -> Product/2

== system Transformation_V11/DUT_V5/UnitConversion/ExtAmpConvert3 ==
  Raw : Inport
  Conv_Factor : Inport  Port=2
  Product : Product  OutDataTypeStr=fixdt(1,16,11)
  Amp : Outport
  wires:
  Raw/1 -> Product/1
  Product/1 -> Amp/1
  Conv_Factor/1 -> Product/2

== system Transformation_V11/DUT_V5/UnitConversion/ExtVoltConvert1 ==
  Raw : Inport
  Gain : Gain  Gain=fi(1/4096)  OutMin=0  OutMax=1  OutDataTypeStr=fixdt(0,16)
  Volts : Outport
  wires:
  Raw/1 -> Gain/1
  Gain/1 -> Volts/1

== system Transformation_V11/DUT_V5/UnitConversion/ExtVoltConvert2 ==
  Raw : Inport
  Gain : Gain  Gain=fi(1/4096)  OutMin=0  OutMax=1  OutDataTypeStr=fixdt(0,16)
  Volts : Outport
  wires:
  Gain/1 -> Volts/1
  Raw/1 -> Gain/1

== system Transformation_V11/DUT_V5/UnitConversion/ExtVoltConvert3 ==
  Raw : Inport
  Gain : Gain  Gain=fi(1/4096)  OutMin=0  OutMax=1  OutDataTypeStr=fixdt(0,16)
  Volts : Outport
  wires:
  Raw/1 -> Gain/1
  Gain/1 -> Volts/1

== system Transformation_V11/DUT_V5/UnitConversion/IntVoltConvert ==
  Raw : Inport
  Gain : Gain  Gain=fi(3/4096)  OutMin=0  OutMax=3  OutDataTypeStr=fixdt(0,16)
  Volts : Outport
  wires:
  Raw/1 -> Gain/1
  Gain/1 -> Volts/1

== system Transformation_V11/DUT_V5/UnitConversion/TempConvert ==
  Raw : Inport
  Add : Sum  Inputs=+-
  Constant : Constant  Value=273.15  OutDataTypeStr=fixdt(0,15)  SampleTime=-1
  Gain : Gain  Gain=fi(503.975/4096)  OutMin=0  OutMax=503.975  OutDataTypeStr=fixdt(0,15)
  DegC : Outport
  wires:
  Gain/1 -> Add/1
  Constant/1 -> Add/2
  Add/1 -> DegC/1
  Raw/1 -> Gain/1

== system Transformation_V11/xadc/xadc_plant/AuxChan ==
  Addr : Inport
  Vaux : Inport  Port=2
  Demux : Demux  Outputs=16
  ExtVoltPlant19 : Subsystem
  Multiport Switch1 : MultiPortSwitch  DataPortOrder=Zero-based contiguous  Inputs=16  DiagnosticForDefault=None  zeroidx=on
  Aux_ADC : Outport
  wires:
  ExtVoltPlant19/1(Raw_ADC) -> Demux/1
  Demux/1 -> Multiport Switch1/2
  Demux/3 -> Multiport Switch1/4
  Demux/2 -> Multiport Switch1/3
  Demux/8 -> Multiport Switch1/9
  Demux/12 -> Multiport Switch1/13
  Demux/6 -> Multiport Switch1/7
  Demux/14 -> Multiport Switch1/15
  Demux/4 -> Multiport Switch1/5
  Demux/10 -> Multiport Switch1/11
  Demux/11 -> Multiport Switch1/12
  Demux/13 -> Multiport Switch1/14
  Demux/5 -> Multiport Switch1/6
  Demux/7 -> Multiport Switch1/8
  Vaux/1 -> ExtVoltPlant19/1(Volts)
  Demux/9 -> Multiport Switch1/10
  Multiport Switch1/1 -> Aux_ADC/1
  Demux/15 -> Multiport Switch1/16
  Addr/1 -> Multiport Switch1/1
  Demux/16 -> Multiport Switch1/17

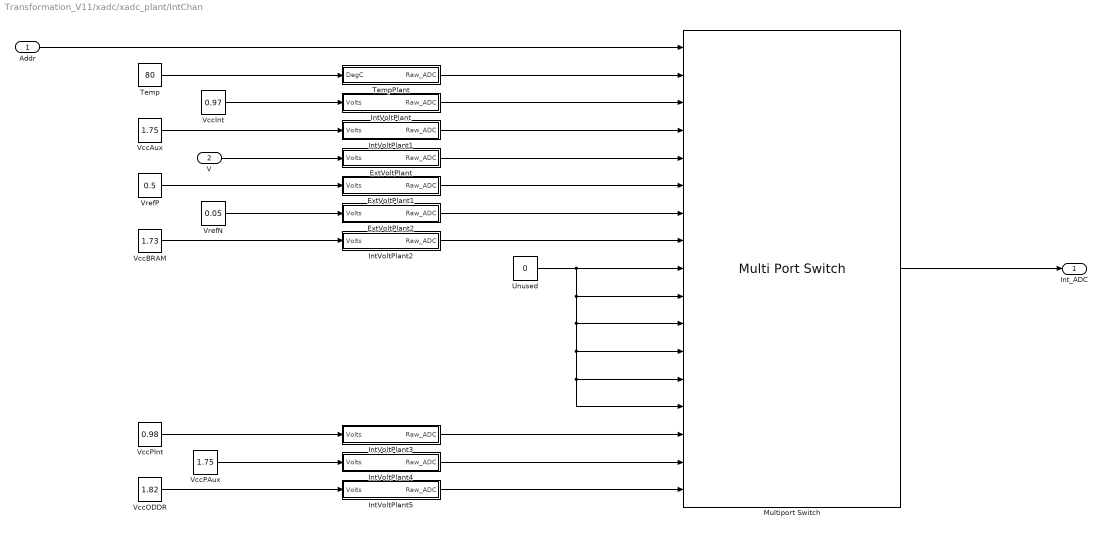
== system Transformation_V11/xadc/xadc_plant/IntChan ==
  Addr : Inport
  V : Inport  Port=2
  ExtVoltPlant : Subsystem
  ExtVoltPlant1 : Subsystem
  ExtVoltPlant2 : Subsystem
  IntVoltPlant : Subsystem
  IntVoltPlant1 : Subsystem
  IntVoltPlant2 : Subsystem
  IntVoltPlant3 : Subsystem
  IntVoltPlant4 : Subsystem
  IntVoltPlant5 : Subsystem
  Multiport Switch : MultiPortSwitch  DataPortOrder=Zero-based contiguous  Inputs=16  DiagnosticForDefault=None  zeroidx=on
  Temp : Constant  Value=80  SampleTime=-1
  TempPlant : Subsystem
  Unused : Constant  Value=0  OutDataTypeStr=Inherit: Inherit via back propagation  SampleTime=-1
  VccAux : Constant  Value=1.75  SampleTime=-1
  VccBRAM : Constant  Value=1.73  SampleTime=-1
  VccInt : Constant  Value=0.97  SampleTime=-1
  VccODDR : Constant  Value=1.82  SampleTime=-1
  VccPAux : Constant  Value=1.75  SampleTime=-1
  VccPInt : Constant  Value=0.98  SampleTime=-1
  VrefN : Constant  Value=0.05  SampleTime=-1
  VrefP : Constant  Value=0.5  SampleTime=-1
  Int_ADC : Outport
  wires:
  IntVoltPlant2/1(Raw_ADC) -> Multiport Switch/8
  VccODDR/1 -> IntVoltPlant5/1(Volts)
  VrefN/1 -> ExtVoltPlant2/1(Volts)
  IntVoltPlant5/1(Raw_ADC) -> Multiport Switch/17
  V/1 -> ExtVoltPlant/1(Volts)
  ExtVoltPlant2/1(Raw_ADC) -> Multiport Switch/7
  TempPlant/1(Raw_ADC) -> Multiport Switch/2
  VccInt/1 -> IntVoltPlant/1(Volts)
  IntVoltPlant4/1(Raw_ADC) -> Multiport Switch/16
  Temp/1 -> TempPlant/1(DegC)
  ExtVoltPlant/1(Raw_ADC) -> Multiport Switch/5
  VccPAux/1 -> IntVoltPlant4/1(Volts)
  VccPInt/1 -> IntVoltPlant3/1(Volts)
  VccAux/1 -> IntVoltPlant1/1(Volts)
  VccBRAM/1 -> IntVoltPlant2/1(Volts)
  IntVoltPlant3/1(Raw_ADC) -> Multiport Switch/15
  Addr/1 -> Multiport Switch/1
  Multiport Switch/1 -> Int_ADC/1
  IntVoltPlant/1(Raw_ADC) -> Multiport Switch/3
  Unused/1 -> Multiport Switch/9, Multiport Switch/14, Multiport Switch/13, Multiport Switch/12, Multiport Switch/11, Multiport Switch/10
  IntVoltPlant1/1(Raw_ADC) -> Multiport Switch/4
  ExtVoltPlant1/1(Raw_ADC) -> Multiport Switch/6
  VrefP/1 -> ExtVoltPlant1/1(Volts)

== system Transformation_V11/xadc/xadc_plant/AuxChan/ExtVoltPlant19 ==
  Volts : Inport
  Bit Concat : hdlsllib/Logic and Bit Operations/Bit Concat  numInputs=2
      settings: SourceProductName=HDL Coder  SourceProductBaseCode=HD
  Data Type Conversion : DataTypeConversion  OutDataTypeStr=fixdt(0,12,0)
  Gain : Gain  Gain=4096
  LSB : Constant  Value=fi(0,0,4,0)  SampleTime=-1
  Raw_ADC : Outport
  wires:
  Bit Concat/1 -> Raw_ADC/1
  LSB/1 -> Bit Concat/2
  Data Type Conversion/1 -> Bit Concat/1
  Volts/1 -> Gain/1
  Gain/1 -> Data Type Conversion/1

== system Transformation_V11/xadc/xadc_plant/IntChan/ExtVoltPlant ==
  Volts : Inport
  Bit Concat : hdlsllib/Logic and Bit Operations/Bit Concat  numInputs=2
      settings: SourceProductName=HDL Coder  SourceProductBaseCode=HD
  Data Type Conversion : DataTypeConversion  OutDataTypeStr=fixdt(0,12,0)
  Gain : Gain  Gain=4096
  LSB : Constant  Value=fi(0,0,4,0)  SampleTime=-1
  Raw_ADC : Outport
  wires:
  Bit Concat/1 -> Raw_ADC/1
  LSB/1 -> Bit Concat/2
  Data Type Conversion/1 -> Bit Concat/1
  Volts/1 -> Gain/1
  Gain/1 -> Data Type Conversion/1

== system Transformation_V11/xadc/xadc_plant/IntChan/ExtVoltPlant1 ==
  Volts : Inport
  Bit Concat : hdlsllib/Logic and Bit Operations/Bit Concat  numInputs=2
      settings: SourceProductName=HDL Coder  SourceProductBaseCode=HD
  Data Type Conversion : DataTypeConversion  OutDataTypeStr=fixdt(0,12,0)
  Gain : Gain  Gain=4096
  LSB : Constant  Value=fi(0,0,4,0)  SampleTime=-1
  Raw_ADC : Outport
  wires:
  Gain/1 -> Data Type Conversion/1
  Volts/1 -> Gain/1
  Data Type Conversion/1 -> Bit Concat/1
  LSB/1 -> Bit Concat/2
  Bit Concat/1 -> Raw_ADC/1

== system Transformation_V11/xadc/xadc_plant/IntChan/ExtVoltPlant2 ==
  Volts : Inport
  Bit Concat : hdlsllib/Logic and Bit Operations/Bit Concat  numInputs=2
      settings: SourceProductName=HDL Coder  SourceProductBaseCode=HD
  Data Type Conversion : DataTypeConversion  OutDataTypeStr=fixdt(0,12,0)
  Gain : Gain  Gain=4096
  LSB : Constant  Value=fi(0,0,4,0)  SampleTime=-1
  Raw_ADC : Outport
  wires:
  Bit Concat/1 -> Raw_ADC/1
  LSB/1 -> Bit Concat/2
  Data Type Conversion/1 -> Bit Concat/1
  Volts/1 -> Gain/1
  Gain/1 -> Data Type Conversion/1

== system Transformation_V11/xadc/xadc_plant/IntChan/IntVoltPlant ==
  Volts : Inport
  Bit Concat : hdlsllib/Logic and Bit Operations/Bit Concat  numInputs=2
      settings: SourceProductName=HDL Coder  SourceProductBaseCode=HD
  Data Type Conversion : DataTypeConversion  OutDataTypeStr=fixdt(0,12,0)
  Gain : Gain  Gain=4096/3
  LSB : Constant  Value=fi(0,0,4,0)  SampleTime=-1
  Raw_ADC : Outport
  wires:
  Gain/1 -> Data Type Conversion/1
  Volts/1 -> Gain/1
  Data Type Conversion/1 -> Bit Concat/1
  LSB/1 -> Bit Concat/2
  Bit Concat/1 -> Raw_ADC/1

== system Transformation_V11/xadc/xadc_plant/IntChan/IntVoltPlant1 ==
  Volts : Inport
  Bit Concat : hdlsllib/Logic and Bit Operations/Bit Concat  numInputs=2
      settings: SourceProductName=HDL Coder  SourceProductBaseCode=HD
  Data Type Conversion : DataTypeConversion  OutDataTypeStr=fixdt(0,12,0)
  Gain : Gain  Gain=4096/3
  LSB : Constant  Value=fi(0,0,4,0)  SampleTime=-1
  Raw_ADC : Outport
  wires:
  Bit Concat/1 -> Raw_ADC/1
  LSB/1 -> Bit Concat/2
  Data Type Conversion/1 -> Bit Concat/1
  Volts/1 -> Gain/1
  Gain/1 -> Data Type Conversion/1

== system Transformation_V11/xadc/xadc_plant/IntChan/IntVoltPlant2 ==
  Volts : Inport
  Bit Concat : hdlsllib/Logic and Bit Operations/Bit Concat  numInputs=2
      settings: SourceProductName=HDL Coder  SourceProductBaseCode=HD
  Data Type Conversion : DataTypeConversion  OutDataTypeStr=fixdt(0,12,0)
  Gain : Gain  Gain=4096/3
  LSB : Constant  Value=fi(0,0,4,0)  SampleTime=-1
  Raw_ADC : Outport
  wires:
  Gain/1 -> Data Type Conversion/1
  Volts/1 -> Gain/1
  Data Type Conversion/1 -> Bit Concat/1
  LSB/1 -> Bit Concat/2
  Bit Concat/1 -> Raw_ADC/1

== system Transformation_V11/xadc/xadc_plant/IntChan/IntVoltPlant3 ==
  Volts : Inport
  Bit Concat : hdlsllib/Logic and Bit Operations/Bit Concat  numInputs=2
      settings: SourceProductName=HDL Coder  SourceProductBaseCode=HD
  Data Type Conversion : DataTypeConversion  OutDataTypeStr=fixdt(0,12,0)
  Gain : Gain  Gain=4096/3
  LSB : Constant  Value=fi(0,0,4,0)  SampleTime=-1
  Raw_ADC : Outport
  wires:
  Bit Concat/1 -> Raw_ADC/1
  LSB/1 -> Bit Concat/2
  Data Type Conversion/1 -> Bit Concat/1
  Volts/1 -> Gain/1
  Gain/1 -> Data Type Conversion/1

== system Transformation_V11/xadc/xadc_plant/IntChan/IntVoltPlant4 ==
  Volts : Inport
  Bit Concat : hdlsllib/Logic and Bit Operations/Bit Concat  numInputs=2
      settings: SourceProductName=HDL Coder  SourceProductBaseCode=HD
  Data Type Conversion : DataTypeConversion  OutDataTypeStr=fixdt(0,12,0)
  Gain : Gain  Gain=4096/3
  LSB : Constant  Value=fi(0,0,4,0)  SampleTime=-1
  Raw_ADC : Outport
  wires:
  Gain/1 -> Data Type Conversion/1
  Volts/1 -> Gain/1
  Data Type Conversion/1 -> Bit Concat/1
  LSB/1 -> Bit Concat/2
  Bit Concat/1 -> Raw_ADC/1

== system Transformation_V11/xadc/xadc_plant/IntChan/IntVoltPlant5 ==
  Volts : Inport
  Bit Concat : hdlsllib/Logic and Bit Operations/Bit Concat  numInputs=2
      settings: SourceProductName=HDL Coder  SourceProductBaseCode=HD
  Data Type Conversion : DataTypeConversion  OutDataTypeStr=fixdt(0,12,0)
  Gain : Gain  Gain=4096/3
  LSB : Constant  Value=fi(0,0,4,0)  SampleTime=-1
  Raw_ADC : Outport
  wires:
  Bit Concat/1 -> Raw_ADC/1
  LSB/1 -> Bit Concat/2
  Data Type Conversion/1 -> Bit Concat/1
  Volts/1 -> Gain/1
  Gain/1 -> Data Type Conversion/1

== system Transformation_V11/xadc/xadc_plant/IntChan/TempPlant ==
  DegC : Inport
  Add : Sum
  Bit Concat : hdlsllib/Logic and Bit Operations/Bit Concat  numInputs=2
      settings: SourceProductName=HDL Coder  SourceProductBaseCode=HD
  Data Type Conversion : DataTypeConversion  OutDataTypeStr=fixdt(0,12,0)
  Gain : Gain  Gain=4096/503.975
  LSB : Constant  Value=fi(0,0,4,0)  SampleTime=-1
  Offset : Constant  Value=273.15  SampleTime=-1
  Raw_ADC : Outport
  wires:
  Offset/1 -> Add/2
  DegC/1 -> Add/1
  Add/1 -> Gain/1
  Data Type Conversion/1 -> Bit Concat/1
  LSB/1 -> Bit Concat/2
  Gain/1 -> Data Type Conversion/1
  Bit Concat/1 -> Raw_ADC/1
